simulink model "TST_WordRequirements"  (Simulink 7.8)
settings: Solver=FixedStepDiscrete  StartTime=0.0  StopTime=10.0  FixedStep=0.02  RelTol=1e-3
settings Model: Creator=kharthforeign  LastModifiedBy=kharthforeign  BufferReuse=off
settings DataIOCC: SaveOutput=off  SignalLogging=off  SaveTime=off
settings OptimizationCC: BlockReduction=off  ConditionallyExecuteInputs=off  OptimizeBlockIOStorage=off  BufferReuse=off  ExpressionFolding=off  LocalBlockOutputs=off  InitFltsAndDblsToZero=on
settings DebuggingCC: FcnCallInpInsideContextMsg=Use local settings  StrictBusMsg=Warning

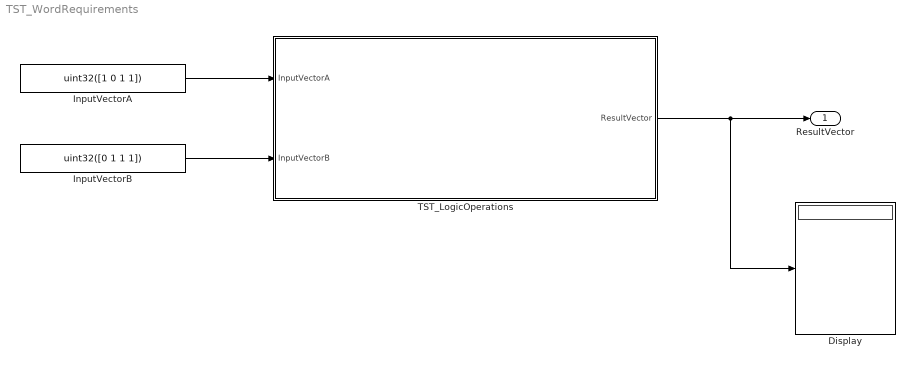
== system TST_WordRequirements ==
  Display : Display
  InputVectorA : Constant  Value=uint32([1 0 1 1])
  InputVectorB : Constant  Value=uint32([0 1 1 1])
  TST_LogicOperations : Subsystem  RequirementInfo={} %GIDa_611058af_54f9_4307_b99e_3d68e731bf77  TreatAsAtomicUnit=on
  ResultVector : Outport
  wires:
  TST_LogicOperations/1(ResultVector) -> ResultVector/1, Display/1
  InputVectorA/1 -> TST_LogicOperations/1(InputVectorA)
  InputVectorB/1 -> TST_LogicOperations/2(InputVectorB)

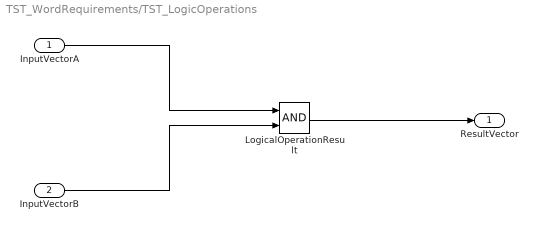
== system TST_WordRequirements/TST_LogicOperations ==
  InputVectorA : Inport
  InputVectorB : Inport  Port=2
  LogicalOperationResult : Logic  RequirementInfo={} %GIDa_cd8a7865_673e_4392_a46c_99735584f465  AllPortsSameDT=off  OutDataTypeStr=boolean
  ResultVector : Outport
  wires:
  InputVectorA/1 -> LogicalOperationResult/1
  InputVectorB/1 -> LogicalOperationResult/2
  LogicalOperationResult/1 -> ResultVector/1
